simulink model "simTwoLinkFDIbasisComparison"  (R2014b)
settings: Solver=ode45  StartTime=0.0  StopTime=tof  FixedStep=dt  MaxStep=dtmax  RelTol=1e-3
values from neighbouring files (symbols this model uses):
  As = zeros(nofstates,nofstates)    [threeLinkFTC.m]    (also in twoLinkFDIbasisComparison.m; twoLinkFTC.m; twoLinkFTCwAdaptive.m)
  c1 = 0    [robotArmWith2Links.m]    (also in twoLinkFDIbasisComparison.m = 1; twoLinkFTC.m; twoLinkFTCwAdaptive.m)
  c2 = 0    [robotArmWith2Links.m]    (also in twoLinkFDIbasisComparison.m = 1; twoLinkFTC.m; twoLinkFTCwAdaptive.m)
  Dhat0 = zeros(6,1)    [threeLinkFTC.m]    (also in twoLinkFDIbasisComparison.m = zeros(4,1); twoLinkFTC.m = zeros(4,1); twoLinkFTCwAdaptive.m = zeros(4,1))
  dtFc = 1*dtmax    (= 0.001)    [threeLinkFTC.m]    (also in twoLinkFDIbasisComparison.m; twoLinkFTC.m; twoLinkFTCwAdaptive.m)
  epsilontheta = 0.01    [threeLinkFTC.m]    (also in twoLinkFDIbasisComparison.m; twoLinkFTC.m; twoLinkFTCwAdaptive.m)
  fault_gamma = 1    [twoLinkFDIbasisComparison.m]
  fault_taumax = 15    [twoLinkFDIbasisComparison.m]
  faultyArm = 3    [threeLinkFTC.m]    (also in twoLinkFDIbasisComparison.m = 2; twoLinkFTC.m = 2; twoLinkFTCwAdaptive.m = 1)
  g = 9.81    [robotArmWith2Links.m]    (also in threeLinkFTC.m; twoLinkFDIbasisComparison.m; twoLinkFTC.m; twoLinkFTCwAdaptive.m)
  GammaW = 1000    [threeLinkFTC.m]    (also in twoLinkFDIbasisComparison.m; twoLinkFTC.m; twoLinkFTCwAdaptive.m)
  I1 = 8.33e-2    (= 0.0833)    [robotArmWith2Links.m]    (also in threeLinkFTC.m = 0.0833333333333; twoLinkFDIbasisComparison.m = 0.0833333333333; twoLinkFTC.m = 0.0833333333333; twoLinkFTCwAdaptive.m = 0.0833333333333)
  I2 = 8.33e-2    (= 0.0833)    [robotArmWith2Links.m]    (also in threeLinkFTC.m = 0.0833333333333; twoLinkFDIbasisComparison.m = 0.0833333333333; twoLinkFTC.m = 0.0833333333333; twoLinkFTCwAdaptive.m = 0.0833333333333)
  ifault = 2    [threeLinkFTC.m]    (also in twoLinkFDIbasisComparison.m; twoLinkFTC.m; twoLinkFTCwAdaptive.m)
  Kp = wn^2    (= 157.913670417)    [threeLinkFTC.m]    (also in twoLinkFDIbasisComparison.m = 3947.84176044; twoLinkFTC.m = 3947.84176044; twoLinkFTCwAdaptive.m = 3947.84176044)
  Kv = 2*ksi*wn    (= 17.5929188601)    [threeLinkFTC.m]    (also in twoLinkFDIbasisComparison.m = 125.663706144; twoLinkFTC.m = 125.663706144; twoLinkFTCwAdaptive.m = 125.663706144)
  l1 = 1    [robotArmWith2Links.m]    (also in threeLinkFTC.m; twoLinkFDIbasisComparison.m; twoLinkFTC.m; twoLinkFTCwAdaptive.m)
  l2 = 1    [robotArmWith2Links.m]    (also in threeLinkFTC.m; twoLinkFDIbasisComparison.m; twoLinkFTC.m; twoLinkFTCwAdaptive.m)
  lc1 = l1/2    (= 0.5)    [robotArmWith2Links.m]    (also in threeLinkFTC.m; twoLinkFDIbasisComparison.m; twoLinkFTC.m; twoLinkFTCwAdaptive.m)
  lc2 = l2/2    (= 0.5)    [robotArmWith2Links.m]    (also in threeLinkFTC.m; twoLinkFDIbasisComparison.m; twoLinkFTC.m; twoLinkFTCwAdaptive.m)
  m1 = 1    [robotArmWith2Links.m]    (also in threeLinkFTC.m; twoLinkFDIbasisComparison.m; twoLinkFTC.m; twoLinkFTCwAdaptive.m)
  m2 = 1    [robotArmWith2Links.m]    (also in threeLinkFTC.m; twoLinkFDIbasisComparison.m; twoLinkFTC.m; twoLinkFTCwAdaptive.m)
  nCheby = 4    [threeLinkFTC.m]    (also in twoLinkFDIbasisComparison.m; twoLinkFTC.m; twoLinkFTCwAdaptive.m)
  nRBF = length(x1is)*length(x2is)*length(x3is)*length(x4is)    [twoLinkFDIbasisComparison.m]
  Ps = lyap(As(4:6,4:6)',Q)    [threeLinkFTC.m]    (also in twoLinkFDIbasisComparison.m = lyap(As(3:4,3:4)',Q); twoLinkFTC.m = lyap(As(3:4,3:4)',Q); twoLinkFTCwAdaptive.m = lyap(As(3:4,3:4)',Q))
  q0 = [80 20]'*pi/180    [robotArmWith2Links.m]    (also in threeLinkFTC.m = [90 0 0]'*pi/180; twoLinkFDIbasisComparison.m = [90 0]'*pi/180; twoLinkFTC.m = [90 0]'*pi/180; twoLinkFTCwAdaptive.m = [90 0]'*pi/180)
  qdot0 = [0 0]'    [robotArmWith2Links.m]    (also in threeLinkFTC.m = [0 0 0]'*pi/180; twoLinkFDIbasisComparison.m = [0 0]'*pi/180; twoLinkFTC.m = [0 0]'*pi/180; twoLinkFTCwAdaptive.m = [0 0]'*pi/180)
  tfault = 5    [threeLinkFTC.m]    (also in twoLinkFDIbasisComparison.m; twoLinkFTC.m; twoLinkFTCwAdaptive.m = 1)
  visualFlag = 0    [robotArmWith2Links.m]    (also in twoLinkFDIbasisComparison.m; twoLinkFTC.m; twoLinkFTCwAdaptive.m)
  visualizationDataFlag = 1    [robotArmWith2Links.m]    (also in twoLinkFDIbasisComparison.m; twoLinkFTC.m; twoLinkFTCwAdaptive.m)
  W0 = 0    [threeLinkFTC.m]    (also in twoLinkFDIbasisComparison.m; twoLinkFTC.m; twoLinkFTCwAdaptive.m)
  Wbnd = 1000    [threeLinkFTC.m]    (also in twoLinkFDIbasisComparison.m; twoLinkFTC.m; twoLinkFTCwAdaptive.m)
  xhat0 = [q0 ; qdot0]    [threeLinkFTC.m]    (also in twoLinkFDIbasisComparison.m; twoLinkFTC.m; twoLinkFTCwAdaptive.m)
  xu = zeros(nRBF,2)    [twoLinkFDIbasisComparison.m]
undefined symbols (not defined in the file or in its folder): Intmax, Intmin, twolinkplot
libraries: simulink x4, vrlib x4, dspbuff3 x2
(part 1 of 2)
settings Model: Creator=alp.marangoz  LastModifiedBy=alpmarangoz
settings SolverCC: AutoInsertRateTranBlk=on
settings DataIOCC: SignalLoggingSaveFormat=ModelDataLogs
settings OptimizationCC: ExpressionDepthLimit=2147483647
settings DebuggingCC: UnderspecifiedInitializationDetection=Classic  MergeDetectMultiDrivingBlocksExec=none  InheritedTsInSrcMsg=none  CheckMatrixSingularityMsg=error  FcnCallInpInsideContextMsg=UseLocalSettings  StateNameClashWarn=warning
settings GRTTargetCC: CombineOutputUpdateFcns=off  GRTInterface=on

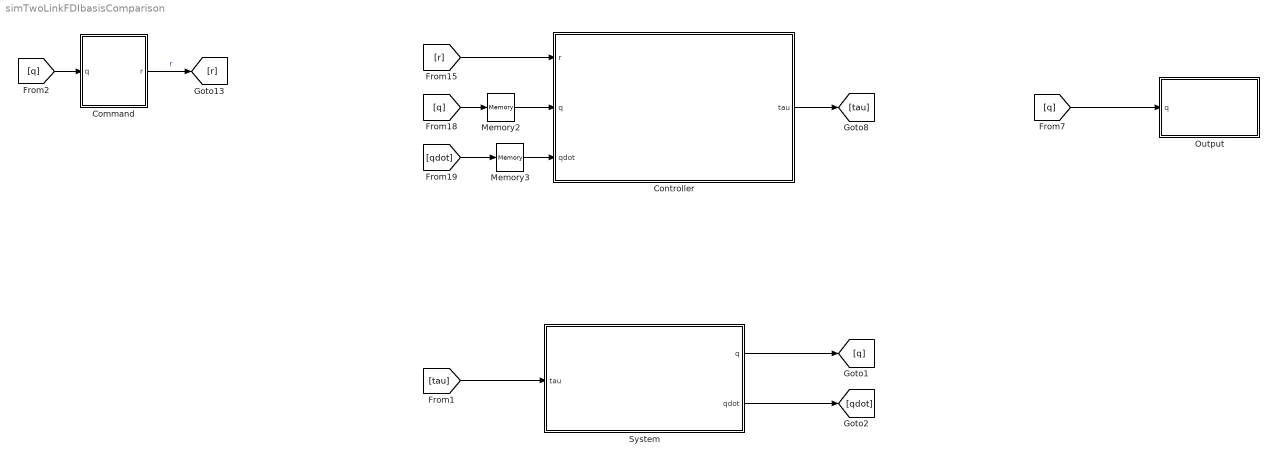
== system simTwoLinkFDIbasisComparison ==
  Command : Subsystem  TreatAsAtomicUnit=on  SystemSampleTime=dtFc
  Controller : Subsystem  TreatAsAtomicUnit=on  SystemSampleTime=dtFc
  Memory2 : Memory  X0=q0  InheritSampleTime=on  LinearizeMemory=on  LinearizeAsDelay=on
  Memory3 : Memory  X0=qdot0  InheritSampleTime=on  LinearizeMemory=on  LinearizeAsDelay=on
  Output : Subsystem  TreatAsAtomicUnit=on
  System : Subsystem  TreatAsAtomicUnit=on
  wires:
  Command/1(r) -> [r]  "r"
  [r] -> Controller/1(r)
  Controller/1(tau) -> [tau]
  [q] -> Output/1(q)
  [tau] -> System/1(tau)
  [q] -> Memory2/1
  [qdot] -> Memory3/1
  System/1(q) -> [q]
  System/2(qdot) -> [qdot]
  [q] -> Command/1(q)
  Memory2/1 -> Controller/2(q)
  Memory3/1 -> Controller/3(qdot)

== system simTwoLinkFDIbasisComparison/Command ==
  q : Inport
  Add1 : Sum  Inputs=-+
  From Workspace : FromWorkspace  VariableName=r  Interpolate=off  OutputAfterFinalValue=Setting to zero
  Memory2 : Memory  X0=q0  InheritSampleTime=on  LinearizeMemory=on  LinearizeAsDelay=on
  Reshape1 : Reshape  OutputDimensionality=Column vector (2-D)
  Terminator1 : Terminator
  r : Outport  InitialOutput=0
  wires:
  From Workspace/1 -> Reshape1/1
  Reshape1/1 -> r/1, [r]  "r"
  [r] -> Add1/2
  Add1/1 -> Terminator1/1  "e"
  [q] -> Add1/1  "q"
  q/1 -> Memory2/1  "q"
  Memory2/1 -> [q]

== system simTwoLinkFDIbasisComparison/Controller ==
  r : Inport
  q : Inport  Port=2
  qdot : Inport  Port=3
  Disturbance Estimator : Subsystem
  Gain : Gain  Gain=-1
  Get System Parameters : Subsystem
  Nominal Controller : Subsystem
  Terminator1 : Terminator
  Terminator2 : Terminator
  tau : Outport
  wires:
  r/1 -> [r]  "r"
  qdot/1 -> [qdot]  "qdot"
  q/1 -> [q]  "q"
  [tau] -> tau/1  "tau"
  [q] -> Get System Parameters/1(q)
  Nominal Controller/1(tau) -> [tau]
  [r] -> Nominal Controller/1(r)
  [H] -> Nominal Controller/4(H)
  [Phi] -> Nominal Controller/5(Phi)
  [qdot] -> Get System Parameters/2(qdot)
  Get System Parameters/1(H) -> [H]
  Get System Parameters/2(Phi) -> [Phi]
  Get System Parameters/3(Cprime) -> [Cp]
  [q] -> Disturbance Estimator/1(q)
  [qdot] -> Disturbance Estimator/2(qdot)
  [H] -> Disturbance Estimator/4(H)
  [Cp] -> Disturbance Estimator/5(Cp)
  [G] -> Disturbance Estimator/6(G)
  Disturbance Estimator/1(xhat) -> Terminator1/1  "xhat"
  Disturbance Estimator/2(Dhat) -> [Dhat]
  [qdot] -> Nominal Controller/3(qdot)
  [q] -> Nominal Controller/2(q)
  [tau] -> Disturbance Estimator/3(tau)
  Get System Parameters/4(G) -> [G]
  Gain/1 -> Terminator2/1  "Dhat"
  [Dhat] -> Gain/1

== system simTwoLinkFDIbasisComparison/Output ==
  q : Inport
  Constant1 : Constant  Value=visualFlag
  Constant3 : Constant  Value=visualizationDataFlag
  Demux4 : Demux  Outputs=2
  two link visualization : Subsystem
  visualization data out : Subsystem  TreatAsAtomicUnit=on
  wires:
  Constant1/1 -> two link visualization/Enable
  Demux4/1 -> two link visualization/1(tht1 [|rad])
  Demux4/2 -> two link visualization/2(tht2 [rad])
  Constant3/1 -> visualization data out/Enable
  q/1 -> visualization data out/1(tht), Demux4/1

== system simTwoLinkFDIbasisComparison/System ==
  tau : Inport
  Fault Insertion : Subsystem
  Integration : Subsystem  TreatAsAtomicUnit=on
  Memory2 : Memory  X0=q0  InheritSampleTime=on  LinearizeMemory=on  LinearizeAsDelay=on
  Memory4 : Memory  X0=qdot0  InheritSampleTime=on  LinearizeMemory=on  LinearizeAsDelay=on
  Reshape5 : Reshape  OutputDimensionality=Column vector (2-D)
  System Parameters : Subsystem
  q : Outport
  qdot : Outport  Port=2
  wires:
  System Parameters/1(H) -> [H]
  System Parameters/2(Phi) -> [Phi]
  [q] -> Memory2/1
  [qdot] -> Memory4/1
  tau/1 -> Reshape5/1  "tau"
  Reshape5/1 -> [tau]  "tau"
  [q] -> q/1  "q"
  [qdot] -> qdot/1  "qdot"
  [tau] -> Fault Insertion/1(tau)
  [Phi] -> Fault Insertion/2(Phi)
  Fault Insertion/2(lockJoint) -> [lockJoint]
  Memory4/1 -> System Parameters/2(qdot)
  [H] -> Integration/1(H)
  [C] -> Integration/2(C)
  [tau] -> Integration/5(tau)
  [lockJoint] -> Integration/6(lockJoint)
  System Parameters/3(C) -> [C]
  System Parameters/4(G) -> [G]
  [G] -> Integration/3(G)
  [F] -> Integration/4(F)
  Integration/1(q) -> [q]
  Integration/2(qdot) -> [qdot]
  Memory2/1 -> System Parameters/1(q)
  Fault Insertion/1(F) -> [F]

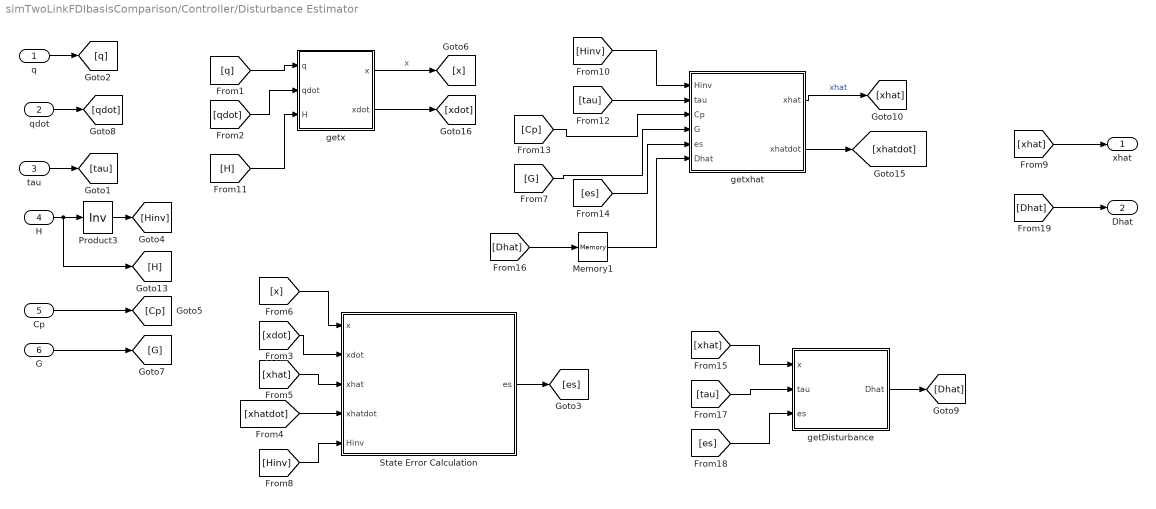
== system simTwoLinkFDIbasisComparison/Controller/Disturbance Estimator ==
  q : Inport
  qdot : Inport  Port=2
  tau : Inport  Port=3
  H : Inport  Port=4
  Cp : Inport  Port=5
  G : Inport  Port=6
  Memory1 : Memory  X0=Dhat0  InheritSampleTime=on  LinearizeMemory=on
  Product3 : Product  Inputs=/  Multiplication=Matrix(*)  RndMeth=Zero
  State Error Calculation : Subsystem
  getDisturbance : Subsystem
  getx : Subsystem
  getxhat : Subsystem
  xhat : Outport
  Dhat : Outport  Port=2
  wires:
  getx/2(xdot) -> [xdot]
  [qdot] -> getx/2(qdot)
  [q] -> getx/1(q)
  Cp/1 -> [Cp]
  Product3/1 -> [Hinv]
  H/1 -> [H], Product3/1
  tau/1 -> [tau]
  [xhat] -> xhat/1
  q/1 -> [q]
  qdot/1 -> [qdot]
  getx/1(x) -> [x]  "x"
  [H] -> getx/3(H)
  [Hinv] -> getxhat/1(Hinv)
  [tau] -> getxhat/2(tau)
  [Cp] -> getxhat/3(Cp)
  [es] -> getxhat/5(es)
  [Dhat] -> Memory1/1
  G/1 -> [G]
  getxhat/1(xhat) -> [xhat]  "xhat"
  getxhat/2(xhatdot) -> [xhatdot]
  [x] -> State Error Calculation/1(x)
  [xdot] -> State Error Calculation/2(xdot)
  [xhat] -> State Error Calculation/3(xhat)
  [xhatdot] -> State Error Calculation/4(xhatdot)
  [Hinv] -> State Error Calculation/5(Hinv)
  State Error Calculation/1(es) -> [es]
  [xhat] -> getDisturbance/1(x)
  [tau] -> getDisturbance/2(tau)
  [es] -> getDisturbance/3(es)
  getDisturbance/1(Dhat) -> [Dhat]
  [Dhat] -> Dhat/1
  Memory1/1 -> getxhat/6(Dhat)
  [G] -> getxhat/4(G)

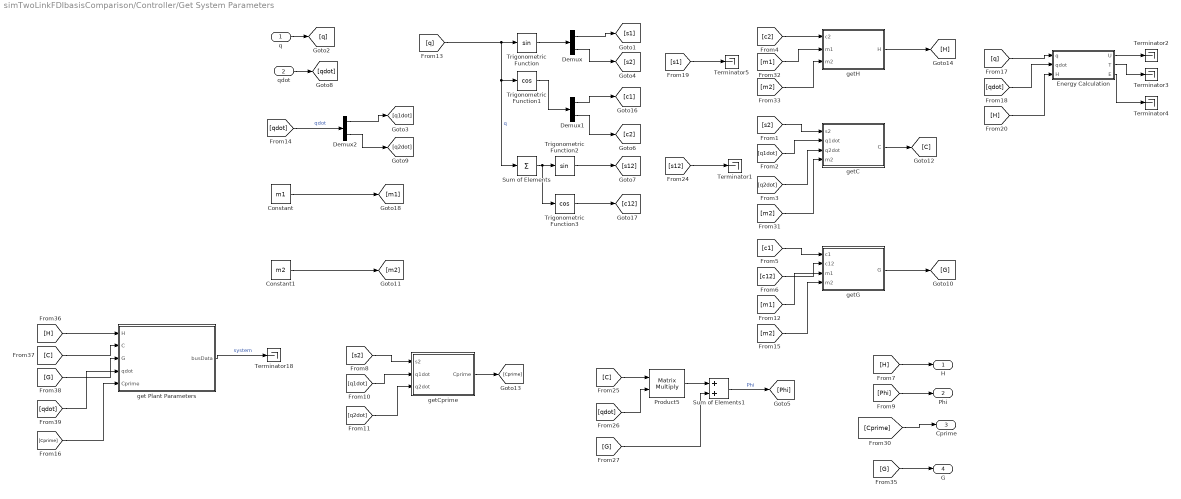
== system simTwoLinkFDIbasisComparison/Controller/Get System Parameters ==
  q : Inport
  qdot : Inport  Port=2
  Constant : Constant  Value=m1
  Constant1 : Constant  Value=m2
  Demux : Demux  Outputs=2
  Demux1 : Demux  Outputs=2
  Demux2 : Demux  Outputs=2
  Energy Calculation : Subsystem
  Product5 : Product  Multiplication=Matrix(*)  RndMeth=Zero
  Sum of Elements : Sum  Inputs=+
  Sum of Elements1 : Sum
  Terminator{1..5,18} (6 alike) : Terminator
  Trigonometric Function : Trigonometry
  Trigonometric Function1 : Trigonometry  Operator=cos
  Trigonometric Function2 : Trigonometry
  Trigonometric Function3 : Trigonometry  Operator=cos
  get Plant Parameters : Subsystem
  getC : Subsystem
  getCprime : Subsystem
  getG : Subsystem
  getH : Subsystem
  H : Outport
  Phi : Outport  Port=2
  Cprime : Outport  Port=3
  G : Outport  Port=4
  wires:
  q/1 -> [q]
  qdot/1 -> [qdot]
  [q] -> Trigonometric Function/1, Trigonometric Function1/1, Sum of Elements/1  "q"
  Trigonometric Function/1 -> Demux/1
  Demux/1 -> [s1]
  Demux/2 -> [s2]
  Demux1/1 -> [c1]
  Demux1/2 -> [c2]
  Trigonometric Function1/1 -> Demux1/1
  Sum of Elements/1 -> Trigonometric Function2/1, Trigonometric Function3/1
  Trigonometric Function2/1 -> [s12]
  [qdot] -> Demux2/1  "qdot"
  Demux2/1 -> [q1dot]
  Demux2/2 -> [q2dot]
  Trigonometric Function3/1 -> [c12]
  [s12] -> Terminator1/1
  [s1] -> Terminator5/1
  [c2] -> getH/1(c2)
  [s2] -> getC/1(s2)
  [q1dot] -> getC/2(q1dot)
  [q2dot] -> getC/3(q2dot)
  getH/1(H) -> [H]
  getC/1(C) -> [C]
  [c1] -> getG/1(c1)
  [c12] -> getG/2(c12)
  getG/1(G) -> [G]
  [q] -> Energy Calculation/1(q)
  [qdot] -> Energy Calculation/2(qdot)
  Energy Calculation/1(U) -> Terminator2/1
  Energy Calculation/2(T) -> Terminator3/1
  Energy Calculation/3(E) -> Terminator4/1
  [H] -> Energy Calculation/3(H)
  [C] -> Product5/1
  [qdot] -> Product5/2
  Product5/1 -> Sum of Elements1/1
  [G] -> Sum of Elements1/2
  Sum of Elements1/1 -> [Phi]  "Phi"
  [H] -> H/1
  [Phi] -> Phi/1
  [s2] -> getCprime/1(s2)
  [q1dot] -> getCprime/2(q1dot)
  [q2dot] -> getCprime/3(q2dot)
  getCprime/1(Cprime) -> [Cprime]
  [Cprime] -> Cprime/1
  [m1] -> getG/3(m1)
  [m2] -> getG/4(m2)
  [m2] -> getC/4(m2)
  [m1] -> getH/2(m1)
  [m2] -> getH/3(m2)
  Constant/1 -> [m1]
  Constant1/1 -> [m2]
  [G] -> G/1
  get Plant Parameters/1(busData) -> Terminator18/1  "system"
  [C] -> get Plant Parameters/2(C)
  [H] -> get Plant Parameters/1(H)
  [G] -> get Plant Parameters/3(G)
  [qdot] -> get Plant Parameters/4(qdot)
  [Cprime] -> get Plant Parameters/5(Cprime)

== system simTwoLinkFDIbasisComparison/Controller/Nominal Controller ==
  r : Inport
  q : Inport  Port=2
  qdot : Inport  Port=3
  H : Inport  Port=4
  Phi : Inport  Port=5
  FBL Controller : Subsystem
  Saturation : Saturate  UpperLimit=2000  LowerLimit=-2000
  tau : Outport
  wires:
  r/1 -> [r]  "r"
  Phi/1 -> [Phi]
  H/1 -> [H]
  [tau] -> Saturation/1  "tau"
  [r] -> FBL Controller/1(r)
  [H] -> FBL Controller/4(H)
  [Phi] -> FBL Controller/5(Phi)
  Saturation/1 -> tau/1
  FBL Controller/1(tau) -> [tau]
  q/1 -> [q]
  qdot/1 -> [qdot]
  [qdot] -> FBL Controller/3(qdot)
  [q] -> FBL Controller/2(q)

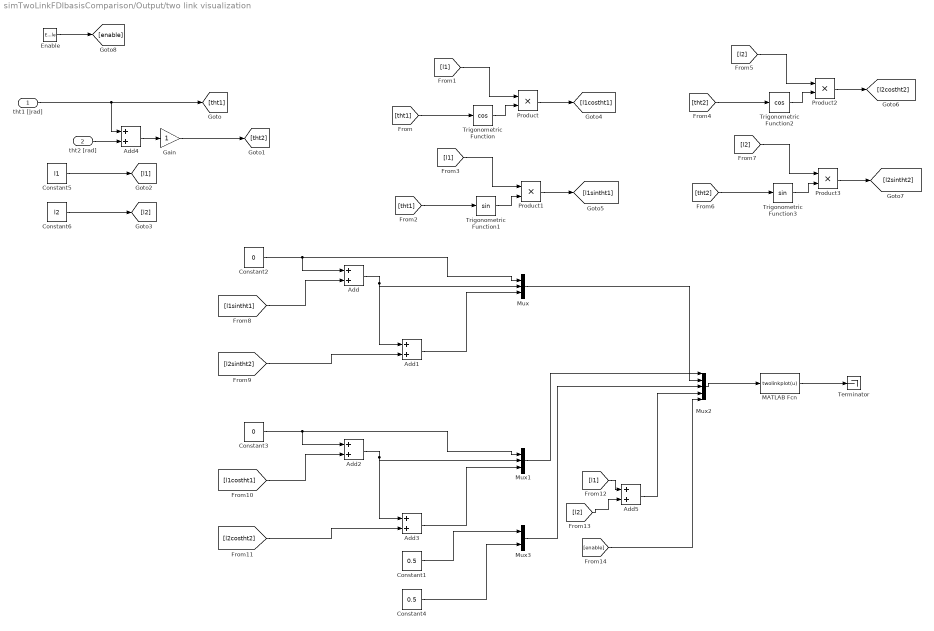
== system simTwoLinkFDIbasisComparison/Output/two link visualization ==
  tht1 [|rad] : Inport
  tht2 [rad] : Inport  Port=2
  Enable : EnablePort  PropagateVarSize=During execution  ShowOutputPort=on
  Add{,1..5} (6 alike) : Sum
  Constant1 : Constant  Value=0.5
  Constant2 : Constant  Value=0
  Constant3 : Constant  Value=0
  Constant4 : Constant  Value=0.5
  Constant5 : Constant  Value=l1  VectorParams1D=off
  Constant6 : Constant  Value=l2  VectorParams1D=off
  Gain : Gain
  MATLAB Fcn : MATLABFcn  MATLABFcn=twolinkplot(u)
  Mux : Mux  Inputs=3
  Mux1 : Mux  Inputs=3
  Mux2 : Mux  Inputs=5
  Mux3 : Mux  Inputs=2
  Product{,1..3} (4 alike) : Product  RndMeth=Zero
  Terminator : Terminator
  Trigonometric Function : Trigonometry  Operator=cos
  Trigonometric Function1 : Trigonometry
  Trigonometric Function2 : Trigonometry  Operator=cos
  Trigonometric Function3 : Trigonometry
  wires:
  [tht1] -> Trigonometric Function/1
  Constant5/1 -> [l1]
  Constant6/1 -> [l2]
  [l1] -> Product/1
  Trigonometric Function/1 -> Product/2
  Product/1 -> [l1costht1]
  [tht1] -> Trigonometric Function1/1
  [l1] -> Product1/1
  Trigonometric Function1/1 -> Product1/2
  Product1/1 -> [l1sintht1]
  [tht2] -> Trigonometric Function2/1
  [l2] -> Product2/1
  Trigonometric Function2/1 -> Product2/2
  Product2/1 -> [l2costht2]
  [tht2] -> Trigonometric Function3/1
  [l2] -> Product3/1
  Trigonometric Function3/1 -> Product3/2
  Product3/1 -> [l2sintht2]
  Constant2/1 -> Add/1, Mux/1
  [l1sintht1] -> Add/2
  Add/1 -> Add1/1, Mux/2
  [l2sintht2] -> Add1/2
  Add1/1 -> Mux/3
  Constant3/1 -> Mux1/1, Add2/1
  [l1costht1] -> Add2/2
  Add2/1 -> Mux1/2, Add3/1
  [l2costht2] -> Add3/2
  Add3/1 -> Mux1/3
  Mux2/1 -> MATLAB Fcn/1
  MATLAB Fcn/1 -> Terminator/1
  tht2 [rad]/1 -> Add4/2
  Gain/1 -> [tht2]
  Add4/1 -> Gain/1
  [l1] -> Add5/1
  [l2] -> Add5/2
  Enable/1 -> [enable]
  Constant1/1 -> Mux3/1
  Constant4/1 -> Mux3/2
  Mux3/1 -> Mux2/3
  Add5/1 -> Mux2/4
  [enable] -> Mux2/5
  tht1 [|rad]/1 -> Add4/1, [tht1]
  Mux1/1 -> Mux2/1
  Mux/1 -> Mux2/2

== system simTwoLinkFDIbasisComparison/Output/visualization data out ==
  tht : Inport
  Enable : EnablePort  PropagateVarSize=During execution
  To Workspace : ToWorkspace  VariableName=thetaForVisualization  SaveFormat=Structure With Time  SampleTime=-1
  wires:
  tht/1 -> To Workspace/1

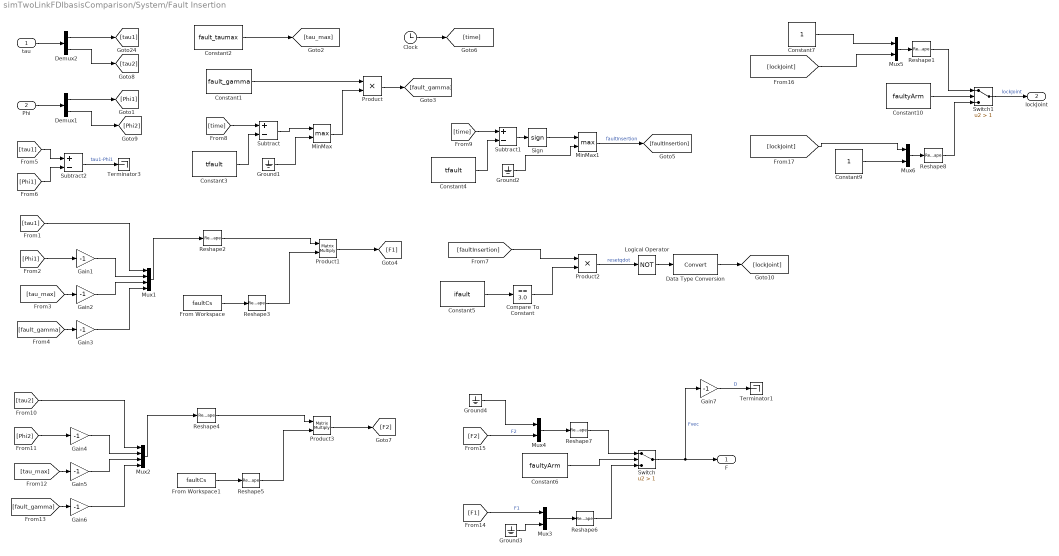
== system simTwoLinkFDIbasisComparison/System/Fault Insertion ==
  tau : Inport
  Phi : Inport  Port=2
  Clock : Clock
  Compare To Constant : simulink/Logic and Bit Operations/Compare To Constant  relop===  const=3.0  OutDataTypeStr=uint8  ZeroCross=off
  Constant1 : Constant  Value=fault_gamma
  Constant10 : Constant  Value=faultyArm  VectorParams1D=off
  Constant2 : Constant  Value=fault_taumax
  Constant3 : Constant  Value=tfault
  Constant4 : Constant  Value=tfault
  Constant5 : Constant  Value=ifault
  Constant6 : Constant  Value=faultyArm  VectorParams1D=off
  Constant7 : Constant
  Constant9 : Constant
  Data Type Conversion : DataTypeConversion
  Demux1 : Demux  Outputs=2
  Demux2 : Demux  Outputs=2
  From Workspace : FromWorkspace  VariableName=faultCs  Interpolate=off  OutputAfterFinalValue=Setting to zero
  From Workspace1 : FromWorkspace  VariableName=faultCs  Interpolate=off  OutputAfterFinalValue=Setting to zero
  Gain{1..7} (7 alike) : Gain  Gain=-1
  Ground{1..4} (4 alike) : Ground
  Logical Operator : Logic  Operator=NOT  AllPortsSameDT=off  OutDataTypeStr=boolean
  MinMax : MinMax  Function=max  Inputs=2
  MinMax1 : MinMax  Function=max  Inputs=2
  Mux1 : Mux
  Mux2 : Mux
  Mux{3..6} (4 alike) : Mux  Inputs=2
  Product : Product  RndMeth=Zero
  Product1 : Product  Multiplication=Matrix(*)  RndMeth=Zero
  Product2 : Product  RndMeth=Zero
  Product3 : Product  Multiplication=Matrix(*)  RndMeth=Zero
  Reshape{1,3,5..8} (6 alike) : Reshape  OutputDimensionality=Column vector (2-D)
  Reshape2 : Reshape  OutputDimensionality=Row vector (2-D)
  Reshape4 : Reshape  OutputDimensionality=Row vector (2-D)
  Sign : Signum
  Subtract : Sum  Inputs=+-
  Subtract1 : Sum  Inputs=+-
  Subtract2 : Sum  Inputs=+-
  Switch : Switch  Criteria=u2 > Threshold  Threshold=1  ZeroCross=off
  Switch1 : Switch  Criteria=u2 > Threshold  Threshold=1  ZeroCross=off
  Terminator1 : Terminator
  Terminator3 : Terminator
  F : Outport
  lockJoint : Outport  Port=2
  wires:
  tau/1 -> Demux2/1
  Phi/1 -> Demux1/1
  Demux2/1 -> [tau1]
  Demux2/2 -> [tau2]
  Demux1/1 -> [Phi1]
  Demux1/2 -> [Phi2]
  Constant2/1 -> [tau_max]
  [tau1] -> Mux1/1
  [Phi1] -> Gain1/1
  [tau_max] -> Gain2/1
  [fault_gamma] -> Gain3/1
  Mux1/1 -> Reshape2/1
  Reshape2/1 -> Product1/1
  [time] -> Subtract/1
  Constant3/1 -> Subtract/2
  Subtract/1 -> MinMax/1
  Ground1/1 -> MinMax/2
  Constant1/1 -> Product/1
  MinMax/1 -> Product/2
  Product/1 -> [fault_gamma]
  From Workspace/1 -> Reshape3/1
  Reshape3/1 -> Product1/2
  Product1/1 -> [F1]
  Gain1/1 -> Mux1/2
  Gain2/1 -> Mux1/3
  Gain3/1 -> Mux1/4
  [time] -> Subtract1/1
  Constant4/1 -> Subtract1/2
  Subtract1/1 -> Sign/1
  Ground2/1 -> MinMax1/2
  Sign/1 -> MinMax1/1
  MinMax1/1 -> [faultInsertion]  "faultInsertion"
  [tau1] -> Subtract2/1
  [Phi1] -> Subtract2/2
  Subtract2/1 -> Terminator3/1  "tau1-Phi1"
  Constant5/1 -> Compare To Constant/1
  [faultInsertion] -> Product2/1
  Compare To Constant/1 -> Product2/2
  Product2/1 -> Logical Operator/1  "resetqdot"
  Logical Operator/1 -> Data Type Conversion/1
  Clock/1 -> [time]
  [tau2] -> Mux2/1
  [Phi2] -> Gain4/1
  [tau_max] -> Gain5/1
  [fault_gamma] -> Gain6/1
  Mux2/1 -> Reshape4/1
  Reshape4/1 -> Product3/1
  From Workspace1/1 -> Reshape5/1
  Reshape5/1 -> Product3/2
  Product3/1 -> [F2]
  Gain4/1 -> Mux2/2
  Gain5/1 -> Mux2/3
  Gain6/1 -> Mux2/4
  Mux3/1 -> Reshape6/1
  Ground3/1 -> Mux3/2
  [F1] -> Mux3/1  "F1"
  Mux4/1 -> Reshape7/1
  [F2] -> Mux4/2  "F2"
  Ground4/1 -> Mux4/1
  Switch/1 -> Gain7/1, F/1  "Fvec"
  Reshape7/1 -> Switch/1
  Reshape6/1 -> Switch/3
  Constant6/1 -> Switch/2
  Mux5/1 -> Reshape1/1
  Data Type Conversion/1 -> [lockJoint]
  Switch1/1 -> lockJoint/1  "lockJoint"
  Mux6/1 -> Reshape8/1
  Constant9/1 -> Mux6/2
  [lockJoint] -> Mux6/1
  Constant7/1 -> Mux5/1
  [lockJoint] -> Mux5/2
  Reshape1/1 -> Switch1/1
  Constant10/1 -> Switch1/2
  Reshape8/1 -> Switch1/3
  Gain7/1 -> Terminator1/1  "D"

== system simTwoLinkFDIbasisComparison/System/Integration ==
  H : Inport
  C : Inport  Port=2
  G : Inport  Port=3
  F : Inport  Port=4
  tau : Inport  Port=5
  lockJoint : Inport  Port=6
  Add : Sum  Inputs=+--
  Constant1 : Constant  Value=2*pi
  Integrator2 : Integrator  InitialCondition=qdot0
  Integrator3 : Integrator  InitialCondition=q0
  Math Function1 : Math  Operator=rem  SaturateOnIntegerOverflow=on
  Product1 : Product  RndMeth=Zero
  Product3 : Product  RndMeth=Zero
  Product4 : Product  Multiplication=Matrix(*)  RndMeth=Zero
  Product5 : Product  Multiplication=Matrix(*)  RndMeth=Zero
  Product6 : Product  Multiplication=Matrix(*)  RndMeth=Zero
  Product7 : Product  Inputs=/  Multiplication=Matrix(*)  RndMeth=Zero
  Reshape : Reshape  OutputDimensionality=Column vector (2-D)
  Reshape3 : Reshape  OutputDimensionality=Column vector (2-D)
  Sum : Sum  Inputs=|+-
  q : Outport
  qdot : Outport  Port=2
  wires:
  lockJoint/1 -> [lockJoint]
  tau/1 -> [tau]
  F/1 -> [F]
  C/1 -> [C]
  H/1 -> Product7/1
  [qdot] -> qdot/1  "qdot"
  [q] -> q/1  "q"
  G/1 -> [G]
  [G] -> Add/2
  [Hinv] -> Product4/1
  Add/1 -> Product4/2
  Product4/1 -> Sum/1
  [Hinv] -> Product5/1
  [C] -> Product5/2
  Product5/1 -> Product6/1
  Product6/1 -> Sum/2
  Integrator3/1 -> Reshape3/1
  Reshape/1 -> Product6/2, Integrator3/1, [qdot]
  Reshape3/1 -> Math Function1/1
  Product7/1 -> [Hinv]
  [tau] -> Add/1
  Constant1/1 -> Math Function1/2
  Math Function1/1 -> [q]  "qr"
  Sum/1 -> Product3/2
  Product3/1 -> Integrator2/1  "qddot"
  [F] -> Add/3
  [lockJoint] -> Product3/1, Product1/1
  Integrator2/1 -> Product1/2
  Product1/1 -> Reshape/1  "qdot"

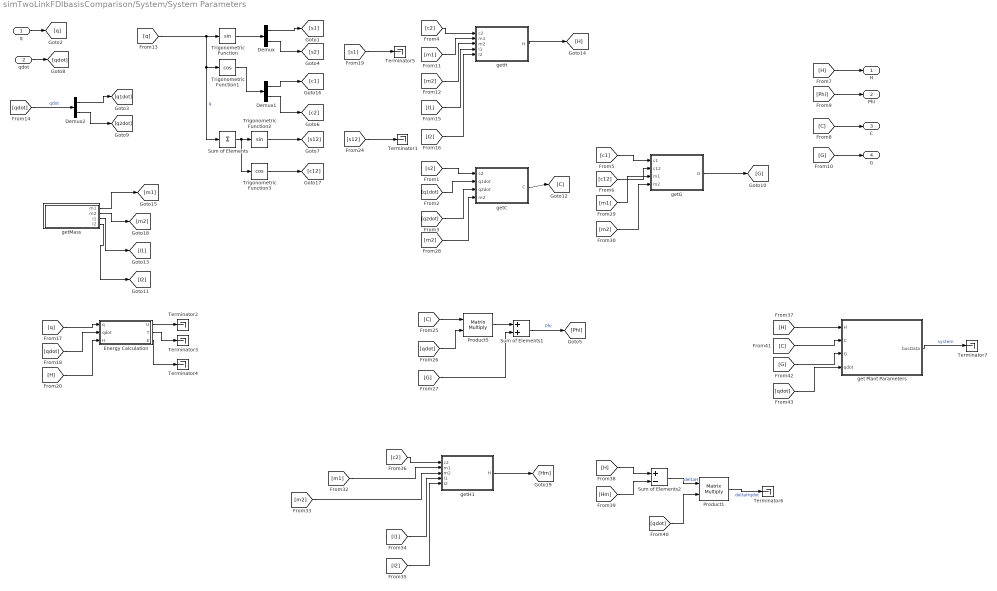
== system simTwoLinkFDIbasisComparison/System/System Parameters ==
  q : Inport
  qdot : Inport  Port=2
  Demux : Demux  Outputs=2
  Demux1 : Demux  Outputs=2
  Demux2 : Demux  Outputs=2
  Energy Calculation : Subsystem
  Product1 : Product  Multiplication=Matrix(*)  RndMeth=Zero
  Product5 : Product  Multiplication=Matrix(*)  RndMeth=Zero
  Sum of Elements : Sum  Inputs=+
  Sum of Elements1 : Sum
  Sum of Elements2 : Sum  Inputs=+-
  Terminator{1..7} (7 alike) : Terminator
  Trigonometric Function : Trigonometry
  Trigonometric Function1 : Trigonometry  Operator=cos
  Trigonometric Function2 : Trigonometry
  Trigonometric Function3 : Trigonometry  Operator=cos
  get Plant Parameters : Subsystem
  getC : Subsystem
  getG : Subsystem
  getH : Subsystem
  getH1 : Subsystem
  getMass : Subsystem
  H : Outport
  Phi : Outport  Port=2
  C : Outport  Port=3
  G : Outport  Port=4
  wires:
  q/1 -> [q]
  qdot/1 -> [qdot]
  [q] -> Trigonometric Function/1, Trigonometric Function1/1, Sum of Elements/1  "q"
  Trigonometric Function/1 -> Demux/1
  Demux/1 -> [s1]
  Demux/2 -> [s2]
  Demux1/1 -> [c1]
  Demux1/2 -> [c2]
  Trigonometric Function1/1 -> Demux1/1
  Sum of Elements/1 -> Trigonometric Function2/1, Trigonometric Function3/1
  Trigonometric Function2/1 -> [s12]
  [qdot] -> Demux2/1  "qdot"
  Demux2/1 -> [q1dot]
  Demux2/2 -> [q2dot]
  Trigonometric Function3/1 -> [c12]
  [s12] -> Terminator1/1
  [s1] -> Terminator5/1
  [c2] -> getH/1(c2)
  [s2] -> getC/1(s2)
  [q1dot] -> getC/2(q1dot)
  [q2dot] -> getC/3(q2dot)
  getH/1(H) -> [H]
  getC/1(C) -> [C]
  [c1] -> getG/1(c1)
  [c12] -> getG/2(c12)
  getG/1(G) -> [G]
  [q] -> Energy Calculation/1(q)
  [qdot] -> Energy Calculation/2(qdot)
  Energy Calculation/1(U) -> Terminator2/1
  Energy Calculation/2(T) -> Terminator3/1
  Energy Calculation/3(E) -> Terminator4/1
  [H] -> Energy Calculation/3(H)
  [C] -> Product5/1
  [qdot] -> Product5/2
  Product5/1 -> Sum of Elements1/1
  [G] -> Sum of Elements1/2
  Sum of Elements1/1 -> [Phi]  "Phi"
  [H] -> H/1
  [Phi] -> Phi/1
  [C] -> C/1
  [G] -> G/1
  [m1] -> getH/2(m1)
  [m2] -> getH/3(m2)
  [I1] -> getH/4(I1)
  [I2] -> getH/5(I2)
  [m2] -> getC/4(m2)
  [m1] -> getG/3(m1)
  [m2] -> getG/4(m2)
  getMass/1(m1) -> [m1]
  getMass/2(m2) -> [m2]
  getMass/3(I1) -> [I1]
  getMass/4(I2) -> [I2]
  [c2] -> getH1/1(c2)
  getH1/1(H) -> [Hm]
  [I1] -> getH1/4(I1)
  [I2] -> getH1/5(I2)
  [H] -> Sum of Elements2/1
  [Hm] -> Sum of Elements2/2
  Sum of Elements2/1 -> Product1/1  "deltaH"
  [qdot] -> Product1/2
  Product1/1 -> Terminator6/1  "deltaHqdot"
  [m2] -> getH1/3(m2)
  [m1] -> getH1/2(m1)
  get Plant Parameters/1(busData) -> Terminator7/1  "system"
  [C] -> get Plant Parameters/2(C)
  [H] -> get Plant Parameters/1(H)
  [G] -> get Plant Parameters/3(G)
  [qdot] -> get Plant Parameters/4(qdot)

== system simTwoLinkFDIbasisComparison/Controller/Disturbance Estimator/State Error Calculation ==
  x : Inport
  xdot : Inport  Port=2
  xhat : Inport  Port=3
  xhatdot : Inport  Port=4
  Hinv : Inport  Port=5
  Add : Sum  Inputs=+-
  Add1 : Sum  Inputs=+-
  Discrete Derivative1 : simulink/Discrete/Discrete Derivative  gainval=1.0  ICPrevScaledInput=0.0  InputProcessing=Inherited  OutMin=[]  OutMax=[]  OutDataType=fixdt(1, 16)  OutScaling=2^-10  RndMeth=Round  DoSatur=off
  Memory1 : Memory  X0=xhat0  InheritSampleTime=on  LinearizeMemory=on  LinearizeAsDelay=on
  Memory4 : Memory  X0=xhat0  InheritSampleTime=on  LinearizeMemory=on  LinearizeAsDelay=on
  Product6 : Product  Multiplication=Matrix(*)  RndMeth=Zero
  Reshape1 : Reshape  OutputDimensionality=Column vector (2-D)
  Reshape2 : Reshape  OutputDimensionality=Column vector (2-D)
  Reshape3 : Reshape  OutputDimensionality=Column vector (2-D)
  Saturation : Saturate  UpperLimit=10  LowerLimit=-10  ZeroCross=off
  Terminator{1..4} (4 alike) : Terminator
  "[1 2]" : Selector  NumberOfDimensions=2  InputPortWidth=3  IndexOptions=Index vector (dialog),Index vector (dialog)  Indices=[1 2],1  OutputSizes=1,1
  "[3 4]" : Selector  NumberOfDimensions=2  InputPortWidth=3  IndexOptions=Index vector (dialog),Index vector (dialog)  Indices=[3 4],1  OutputSizes=1,1
  es : Outport
  wires:
  [Hinv] -> Product6/1
  xdot/1 -> [xdot]
  x/1 -> [x]
  Saturation/1 -> [esdot]  "esdotflt"
  Discrete Derivative1/1 -> Saturation/1  "esdot"
  Reshape2/1 -> [es], Discrete Derivative1/1
  [xhat] -> Memory4/1
  [x] -> Add/2
  Add/1 -> Reshape2/1  "es"
  Memory4/1 -> Add/1
  xhat/1 -> [xhat]
  xhatdot/1 -> [xhatdot]
  Hinv/1 -> [Hinv]
  [xhatdot] -> Memory1/1
  [xdot] -> Add1/2
  Add1/1 -> Reshape1/1  "esdot2"
  Memory1/1 -> Add1/1
  [esdot] -> Terminator3/1
  [es] -> es/1
  [xhat] -> Reshape3/1
  Reshape3/1 -> "[1 2]"/1, "[3 4]"/1
  "[3 4]"/1 -> Product6/2
  "[1 2]"/1 -> Terminator2/1  "qhat"
  Product6/1 -> Terminator1/1  "qhatdot"
  Reshape1/1 -> Terminator4/1

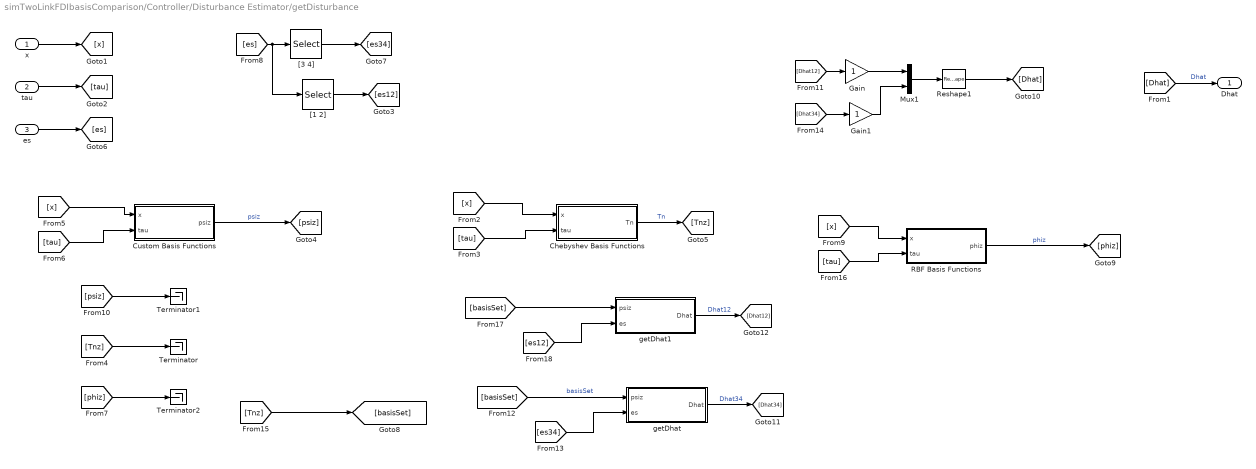
== system simTwoLinkFDIbasisComparison/Controller/Disturbance Estimator/getDisturbance ==
  x : Inport
  tau : Inport  Port=2
  es : Inport  Port=3
  Chebyshev Basis Functions : Subsystem
  Custom Basis Functions : Subsystem
  Gain : Gain
  Gain1 : Gain
  Mux1 : Mux  Inputs=2
  RBF Basis Functions : Subsystem
  Reshape1 : Reshape  OutputDimensionality=Column vector (2-D)
  Terminator : Terminator
  Terminator1 : Terminator
  Terminator2 : Terminator
  "[1 2]" : Selector  NumberOfDimensions=2  InputPortWidth=3  IndexOptions=Index vector (dialog),Index vector (dialog)  Indices=[1 2],1  OutputSizes=1,1
  "[3 4]" : Selector  NumberOfDimensions=2  InputPortWidth=3  IndexOptions=Index vector (dialog),Index vector (dialog)  Indices=[3 4],1  OutputSizes=1,1
  getDhat : Subsystem  TreatAsAtomicUnit=on
  getDhat1 : Subsystem  TreatAsAtomicUnit=on
  Dhat : Outport
  wires:
  [Dhat] -> Dhat/1  "Dhat"
  x/1 -> [x]
  tau/1 -> [tau]
  es/1 -> [es]
  [es] -> "[1 2]"/1, "[3 4]"/1
  "[3 4]"/1 -> [es34]
  [Dhat12] -> Gain/1
  Mux1/1 -> Reshape1/1
  Reshape1/1 -> [Dhat]
  [Dhat34] -> Gain1/1
  [basisSet] -> getDhat/1(psiz)  "basisSet"
  [es34] -> getDhat/2(es)
  getDhat/1(Dhat) -> [Dhat34]  "Dhat34"
  Gain/1 -> Mux1/1
  Gain1/1 -> Mux1/2
  [x] -> Custom Basis Functions/1(x)
  [tau] -> Custom Basis Functions/2(tau)
  Custom Basis Functions/1(psiz) -> [psiz]  "psiz"
  Chebyshev Basis Functions/1(Tn) -> [Tnz]  "Tn"
  [x] -> Chebyshev Basis Functions/1(x)
  [tau] -> Chebyshev Basis Functions/2(tau)
  [Tnz] -> Terminator/1
  [psiz] -> Terminator1/1
  [Tnz] -> [basisSet]
  RBF Basis Functions/1(phiz) -> [phiz]  "phiz"
  [phiz] -> Terminator2/1
  [tau] -> RBF Basis Functions/2(tau)
  [x] -> RBF Basis Functions/1(x)
  [basisSet] -> getDhat1/1(psiz)
  [es12] -> getDhat1/2(es)
  getDhat1/1(Dhat) -> [Dhat12]  "Dhat12"
  "[1 2]"/1 -> [es12]

== system simTwoLinkFDIbasisComparison/Controller/Disturbance Estimator/getx ==
  q : Inport
  qdot : Inport  Port=2
  H : Inport  Port=3
  Demux : Demux  Outputs=2
  Demux1 : Demux  Outputs=2
  Discrete Derivative : simulink/Discrete/Discrete Derivative  gainval=1.0  ICPrevScaledInput=0.0  InputProcessing=Inherited  OutMin=[]  OutMax=[]  OutDataType=fixdt(1, 16)  OutScaling=2^-10  RndMeth=Round  DoSatur=off
  Mux : Mux
  Product6 : Product  Multiplication=Matrix(*)  RndMeth=Zero
  Reshape : Reshape  OutputDimensionality=Column vector (2-D)
  x : Outport
  xdot : Outport  Port=2
  wires:
  Discrete Derivative/1 -> xdot/1  "xdot"
  q/1 -> [q]
  qdot/1 -> [qdot]
  H/1 -> [H]
  [H] -> Product6/1
  [qdot] -> Product6/2
  [q] -> Demux/1
  Product6/1 -> Demux1/1
  Demux/1 -> Mux/1
  Demux/2 -> Mux/2
  Demux1/1 -> Mux/3
  Demux1/2 -> Mux/4
  Mux/1 -> Reshape/1
  Reshape/1 -> x/1, Discrete Derivative/1

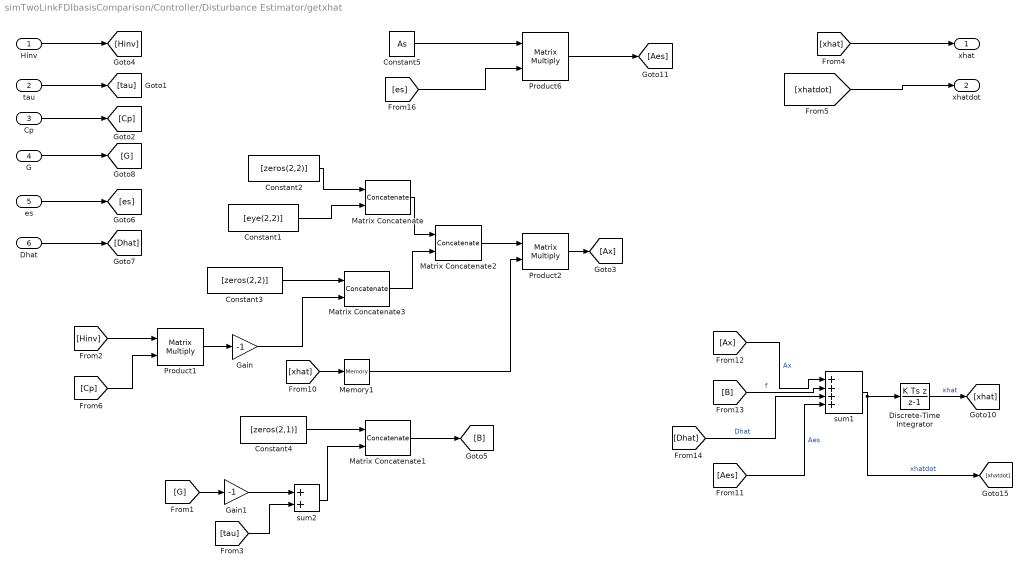
== system simTwoLinkFDIbasisComparison/Controller/Disturbance Estimator/getxhat ==
  Hinv : Inport
  tau : Inport  Port=2
  Cp : Inport  Port=3
  G : Inport  Port=4
  es : Inport  Port=5
  Dhat : Inport  Port=6
  Constant1 : Constant  Value=[eye(2,2)]  VectorParams1D=off
  Constant2 : Constant  Value=[zeros(2,2)]  VectorParams1D=off
  Constant3 : Constant  Value=[zeros(2,2)]
  Constant4 : Constant  Value=[zeros(2,1)]  VectorParams1D=off
  Constant5 : Constant  Value=As
  Discrete-Time Integrator : DiscreteIntegrator  IntegratorMethod=Integration: Backward Euler  InitialCondition=xhat0  InitialConditionSetting=State (most efficient)  SampleTime=-1  UpperSaturationLimit=Intmax  LowerSaturationLimit=Intmin
  Gain : Gain  Gain=-1
  Gain1 : Gain  Gain=-1
  Matrix Concatenate : Concatenate  Mode=Multidimensional array  ConcatenateDimension=2
  Matrix Concatenate1 : Concatenate  Mode=Multidimensional array
  Matrix Concatenate2 : Concatenate  Mode=Multidimensional array
  Matrix Concatenate3 : Concatenate  Mode=Multidimensional array  ConcatenateDimension=2
  Memory1 : Memory  X0=xhat0  InheritSampleTime=on  LinearizeMemory=on  LinearizeAsDelay=on
  Product1 : Product  Multiplication=Matrix(*)  RndMeth=Zero
  Product2 : Product  Multiplication=Matrix(*)  RndMeth=Zero
  Product6 : Product  Multiplication=Matrix(*)  RndMeth=Zero
  sum1 : Sum  Inputs=++++
  sum2 : Sum
  xhat : Outport
  xhatdot : Outport  Port=2
  wires:
  [Dhat] -> sum1/3  "Dhat"
  [B] -> sum1/2  "f"
  [Ax] -> sum1/1  "Ax"
  [Aes] -> sum1/4  "Aes"
  sum1/1 -> [xhatdot], Discrete-Time Integrator/1  "xhatdot"
  Discrete-Time Integrator/1 -> [xhat]  "xhat"
  Memory1/1 -> Product2/2
  Product2/1 -> [Ax]
  [xhat] -> Memory1/1
  Matrix Concatenate/1 -> Matrix Concatenate2/1
  Constant2/1 -> Matrix Concatenate/1
  Hinv/1 -> [Hinv]
  Matrix Concatenate2/1 -> Product2/1
  tau/1 -> [tau]
  Cp/1 -> [Cp]
  [G] -> Gain1/1
  [tau] -> sum2/2
  Constant4/1 -> Matrix Concatenate1/1
  sum2/1 -> Matrix Concatenate1/2
  Matrix Concatenate1/1 -> [B]
  Product6/1 -> [Aes]
  Constant5/1 -> Product6/1
  [es] -> Product6/2
  es/1 -> [es]
  Dhat/1 -> [Dhat]
  G/1 -> [G]
  Constant1/1 -> Matrix Concatenate/2
  Constant3/1 -> Matrix Concatenate3/1
  Matrix Concatenate3/1 -> Matrix Concatenate2/2
  [Hinv] -> Product1/1
  [Cp] -> Product1/2
  Product1/1 -> Gain/1
  Gain/1 -> Matrix Concatenate3/2
  Gain1/1 -> sum2/1
  [xhat] -> xhat/1
  [xhatdot] -> xhatdot/1

== system simTwoLinkFDIbasisComparison/Controller/Get System Parameters/Energy Calculation ==
  q : Inport
  qdot : Inport  Port=2
  H : Inport  Port=3
  Constant : Constant  Value=l1  VectorParams1D=off
  Constant1 : Constant  Value=l2  VectorParams1D=off
  Demux : Demux  Outputs=2
  Gain : Gain  Gain=1/2
  Gain1 : Gain  Gain=0.5
  Gain5 : Gain  Gain=0.5*m1*g
  Gain6 : Gain  Gain=m2*g
  Math Function : Math  Operator=transpose  SaturateOnIntegerOverflow=on
  Product1 : Product  RndMeth=Zero
  Product3 : Product  RndMeth=Zero
  Product5 : Product  Inputs=3  Multiplication=Matrix(*)  RndMeth=Zero
  Sum of Elements : Sum  Inputs=+
  Sum1 : Sum
  Sum2 : Sum
  Sum3 : Sum
  Terminator4 : Terminator
  Trigonometric Function : Trigonometry
  Trigonometric Function2 : Trigonometry
  U : Outport
  T : Outport  Port=2
  E : Outport  Port=3
  wires:
  [q] -> Trigonometric Function/1, Sum of Elements/1
  Trigonometric Function/1 -> Demux/1
  Demux/1 -> [s1]
  Demux/2 -> Terminator4/1
  Sum of Elements/1 -> Trigonometric Function2/1
  Trigonometric Function2/1 -> [s12]
  [qdot] -> Math Function/1
  Math Function/1 -> Product5/1
  [H] -> Product5/2
  [qdot] -> Product5/3
  Product5/1 -> Gain/1
  [l1sintht1] -> Gain5/1
  Gain/1 -> [T]
  [l1sintht1] -> Sum1/1
  [l2sintht12] -> Gain1/1
  Gain5/1 -> Sum3/1
  Gain6/1 -> Sum3/2
  [T] -> Sum2/1
  [U] -> Sum2/2
  q/1 -> [q]
  qdot/1 -> [qdot]
  Sum2/1 -> E/1  "E"
  [U] -> U/1  "U"
  [T] -> T/1  "T"
  Constant/1 -> Product1/1
  [s1] -> Product1/2
  Product1/1 -> [l1sintht1]
  Constant1/1 -> Product3/1
  [s12] -> Product3/2
  Product3/1 -> [l2sintht12]
  Gain1/1 -> Sum1/2
  Sum1/1 -> Gain6/1
  Sum3/1 -> [U]
  H/1 -> [H]

== system simTwoLinkFDIbasisComparison/Controller/Get System Parameters/get Plant Parameters ==
  H : Inport
  C : Inport  Port=2
  G : Inport  Port=3
  qdot : Inport  Port=4
  Cprime : Inport  Port=5
  {1,5,7,11} (4 alike) : Selector  NumberOfDimensions=2  InputPortWidth=3  IndexOptions=Index vector (dialog),Index vector (dialog)  Indices=1,1  OutputSizes=1,1
  12 : Selector  NumberOfDimensions=2  InputPortWidth=3  IndexOptions=Index vector (dialog),Index vector (dialog)  Indices=1,2  OutputSizes=1,1
  2 : Selector  NumberOfDimensions=2  InputPortWidth=3  IndexOptions=Index vector (dialog),Index vector (dialog)  Indices=1,2  OutputSizes=1,1
  {3,6,8,21} (4 alike) : Selector  NumberOfDimensions=2  InputPortWidth=3  IndexOptions=Index vector (dialog),Index vector (dialog)  Indices=2,1  OutputSizes=1,1
  22 : Selector  NumberOfDimensions=2  InputPortWidth=3  IndexOptions=Index vector (dialog),Index vector (dialog)  Indices=2,2  OutputSizes=1,1
  4 : Selector  NumberOfDimensions=2  InputPortWidth=3  IndexOptions=Index vector (dialog),Index vector (dialog)  Indices=2,2  OutputSizes=1,1
  Bus Creator : BusCreator  Inputs=16
  Product5 : Product  Multiplication=Matrix(*)  RndMeth=Zero
  Sum of Elements1 : Sum
  busData : Outport
  wires:
  [H] -> 11/1, 12/1, 21/1, 22/1
  [C] -> 1/1, 2/1, 4/1, 3/1
  [G] -> 6/1, 5/1
  [C] -> Product5/1
  [qdot] -> Product5/2
  Product5/1 -> Sum of Elements1/1
  [G] -> Sum of Elements1/2
  Sum of Elements1/1 -> 7/1, 8/1
  Bus Creator/1 -> busData/1
  H/1 -> [H]  "H"
  C/1 -> [C]  "C"
  G/1 -> [G]  "G"
  qdot/1 -> [qdot]
  [G] -> Bus Creator/4
  [Cprime] -> Bus Creator/3
  [C] -> Bus Creator/2
  [H] -> Bus Creator/1
  22/1 -> Bus Creator/8  "H22"
  21/1 -> Bus Creator/7  "H21"
  1/1 -> Bus Creator/9  "C11"
  12/1 -> Bus Creator/6  "H12"
  2/1 -> Bus Creator/10  "C12"
  11/1 -> Bus Creator/5  "H11"
  3/1 -> Bus Creator/11  "C21"
  4/1 -> Bus Creator/12  "C22"
  5/1 -> Bus Creator/13  "G_1"
  6/1 -> Bus Creator/14  "G_2"
  7/1 -> Bus Creator/15  "phi1"
  8/1 -> Bus Creator/16  "phi2"
  Cprime/1 -> [Cprime]  "Cprime"

== system simTwoLinkFDIbasisComparison/Controller/Get System Parameters/getC ==
  s2 : Inport
  q1dot : Inport  Port=2
  q2dot : Inport  Port=3
  m2 : Inport  Port=4
  Constant2 : Constant  Value=0  VectorParams1D=off
  Gain4 : Gain  Gain=l1*lc2
  Gain6 : Gain  Gain=-1
  Gain7 : Gain  Gain=-1
  Matrix Concatenate : Concatenate  Mode=Multidimensional array  ConcatenateDimension=2
  Matrix Concatenate1 : Concatenate  Mode=Multidimensional array  ConcatenateDimension=2
  Matrix Concatenate2 : Concatenate  Mode=Multidimensional array
  Product{,8..10} (4 alike) : Product  RndMeth=Zero
  Sum4 : Sum
  C : Outport
  wires:
  s2/1 -> [s2]
  q1dot/1 -> [q1dot]
  q2dot/1 -> [q2dot]
  [C] -> C/1
  [m2] -> Gain4/1
  Gain4/1 -> Product/1
  [s2] -> Product/2
  Product/1 -> [h]
  [h] -> Gain6/1
  [h] -> Gain7/1
  Sum4/1 -> Product10/1
  Gain7/1 -> Product10/2
  Product10/1 -> [C12]
  [q2dot] -> Sum4/2
  Constant2/1 -> [C22]
  [h] -> Product8/2
  [q1dot] -> Product8/1
  Product8/1 -> [C21]
  Gain6/1 -> Product9/2
  Product9/1 -> [C11]
  [q2dot] -> Product9/1
  [q1dot] -> Sum4/1
  Matrix Concatenate2/1 -> [C]
  [C22] -> Matrix Concatenate1/2
  [C21] -> Matrix Concatenate1/1
  Matrix Concatenate1/1 -> Matrix Concatenate2/2
  Matrix Concatenate/1 -> Matrix Concatenate2/1
  [C12] -> Matrix Concatenate/2
  [C11] -> Matrix Concatenate/1
  m2/1 -> [m2]

== system simTwoLinkFDIbasisComparison/Controller/Get System Parameters/getCprime ==
  s2 : Inport
  q1dot : Inport  Port=2
  q2dot : Inport  Port=3
  Constant1 : Constant  Value=0  VectorParams1D=off
  Constant2 : Constant  Value=m2
  Gain1 : Gain  Gain=2
  Gain2 : Gain  Gain=l1*lc2
  Gain4 : Gain  Gain=-1
  Gain6 : Gain  Gain=-3
  Gain7 : Gain  Gain=-1
  Matrix Concatenate : Concatenate  Mode=Multidimensional array  ConcatenateDimension=2
  Matrix Concatenate1 : Concatenate  Mode=Multidimensional array  ConcatenateDimension=2
  Matrix Concatenate2 : Concatenate  Mode=Multidimensional array
  Product{,1,9..10} (4 alike) : Product  RndMeth=Zero
  Sum1 : Sum  Inputs=-+
  Sum4 : Sum
  Cprime : Outport
  wires:
  s2/1 -> [s2]
  q1dot/1 -> [q1dot]
  q2dot/1 -> [q2dot]
  [h] -> Gain6/1
  [h] -> Gain7/1
  Sum4/1 -> Product10/1
  Gain7/1 -> Product10/2
  Product10/1 -> [C12]
  [q2dot] -> Gain1/1
  Constant1/1 -> [C22]
  Gain6/1 -> Product9/2
  Product9/1 -> [C11]
  [q2dot] -> Product9/1
  [q1dot] -> Sum4/1
  Matrix Concatenate2/1 -> Cprime/1
  [C22] -> Matrix Concatenate1/2
  [C21] -> Matrix Concatenate1/1
  Matrix Concatenate1/1 -> Matrix Concatenate2/2
  Matrix Concatenate/1 -> Matrix Concatenate2/1
  [C12] -> Matrix Concatenate/2
  [C11] -> Matrix Concatenate/1
  Gain1/1 -> Sum4/2
  [h] -> Gain4/1
  Sum1/1 -> Product1/1
  Gain4/1 -> Product1/2
  Product1/1 -> [C21]
  [q2dot] -> Sum1/2
  [q1dot] -> Sum1/1
  [m2] -> Gain2/1
  Gain2/1 -> Product/1
  [s2] -> Product/2
  Product/1 -> [h]
  Constant2/1 -> [m2]

== system simTwoLinkFDIbasisComparison/Controller/Get System Parameters/getG ==
  c1 : Inport
  c12 : Inport  Port=2
  m1 : Inport  Port=3
  m2 : Inport  Port=4
  Add1 : Sum
  Add2 : Sum
  Gain10 : Gain  Gain=lc2
  Gain11 : Gain  Gain=g
  Gain2 : Gain
  Gain5 : Gain  Gain=lc1
  Gain6 : Gain  Gain=l1
  Gain7 : Gain  Gain=g
  Gain8 : Gain  Gain=lc2
  Gain9 : Gain  Gain=g
  Matrix Concatenate2 : Concatenate  Mode=Multidimensional array
  Product1 : Product  RndMeth=Zero
  Product2 : Product  RndMeth=Zero
  Product3 : Product  RndMeth=Zero
  G : Outport
  wires:
  c12/1 -> [c12]
  c1/1 -> [c1]
  Matrix Concatenate2/1 -> Gain2/1
  [G11] -> Matrix Concatenate2/1
  [G21] -> Matrix Concatenate2/2
  Gain2/1 -> G/1
  [m1] -> Gain5/1
  Gain5/1 -> Add1/1
  [m2] -> Gain6/1
  Gain6/1 -> Add1/2
  Add1/1 -> Gain7/1
  Gain7/1 -> Product1/1
  [c1] -> Product1/2
  [m2] -> Gain8/1
  Gain8/1 -> Gain9/1
  Gain9/1 -> Product2/1
  [c12] -> Product2/2
  Product1/1 -> Add2/1
  Product2/1 -> Add2/2
  Add2/1 -> [G11]
  [m2] -> Gain10/1
  Gain10/1 -> Gain11/1
  Gain11/1 -> Product3/1
  [c12] -> Product3/2
  Product3/1 -> [G21]
  m1/1 -> [m1]
  m2/1 -> [m2]

== system simTwoLinkFDIbasisComparison/Controller/Get System Parameters/getH ==
  c2 : Inport
  m1 : Inport  Port=2
  m2 : Inport  Port=3
  Constant2 : Constant  Value=I2
  Constant4 : Constant  Value=I1
  Gain : Gain  Gain=2
  Gain1 : Gain  Gain=lc2^2
  Gain4 : Gain  Gain=l1*lc2
  Gain5 : Gain  Gain=lc1^2
  Gain6 : Gain  Gain=l1^2+lc2^2
  Gain7 : Gain  Gain=lc2^2
  Matrix Concatenate : Concatenate  Mode=Multidimensional array  ConcatenateDimension=2
  Matrix Concatenate1 : Concatenate  Mode=Multidimensional array  ConcatenateDimension=2
  Matrix Concatenate2 : Concatenate  Mode=Multidimensional array
  Product : Product  RndMeth=Zero
  Sum : Sum  Inputs=+++++
  Sum1 : Sum  Inputs=+++
  Sum2 : Sum
  H : Outport
  wires:
  [H11] -> Matrix Concatenate/1
  [H12] -> Matrix Concatenate/2
  Matrix Concatenate/1 -> Matrix Concatenate2/1
  Matrix Concatenate1/1 -> Matrix Concatenate2/2
  [H21] -> Matrix Concatenate1/1
  [H22] -> Matrix Concatenate1/2
  Matrix Concatenate2/1 -> H/1
  c2/1 -> [c2]
  Sum/1 -> [H11]
  Sum1/1 -> [H12], [H21]
  [m2] -> Gain4/1
  Gain4/1 -> Product/1
  [c2] -> Product/2
  Product/1 -> [a]
  [m1] -> Gain5/1
  [m2] -> Gain6/1
  [I1] -> Sum/1
  [I2] -> Sum/2
  Gain5/1 -> Sum/3
  [a] -> Gain/1
  Gain6/1 -> Sum/4
  Gain/1 -> Sum/5
  [m2] -> Gain7/1
  [I2] -> Sum1/1
  Gain7/1 -> Sum1/2
  [a] -> Sum1/3
  [m2] -> Gain1/1
  [I2] -> Sum2/1
  Gain1/1 -> Sum2/2
  Sum2/1 -> [H22]
  Constant4/1 -> [I1]
  Constant2/1 -> [I2]
  m1/1 -> [m1]
  m2/1 -> [m2]

== system simTwoLinkFDIbasisComparison/Controller/Nominal Controller/FBL Controller ==
  r : Inport
  q : Inport  Port=2
  qdot : Inport  Port=3
  H : Inport  Port=4
  Phi : Inport  Port=5
  Add : Sum  Inputs=-+
  Add1 : Sum  Inputs=-+
  Add2 : Sum
  Add3 : Sum
  Add4 : Sum
  Constant2 : Constant  Value=[0 0]'
  Discrete Derivative : simulink/Discrete/Discrete Derivative  gainval=1.0  ICPrevScaledInput=0.0  InputProcessing=Inherited  OutMin=[]  OutMax=[]  OutDataType=fixdt(1, 16)  OutScaling=2^-10  DoSatur=off
  Gain : Gain  Gain=-Kv
  Gain1 : Gain  Gain=-Kp
  Product2 : Product  Multiplication=Matrix(*)  RndMeth=Zero
  Saturation : Saturate  UpperLimit=10  LowerLimit=-10
  tau : Outport
  wires:
  [v] -> Product2/2
  Product2/1 -> Add4/1
  [Phi] -> Add4/2
  [H] -> Product2/1
  [r] -> Add/1
  Add/1 -> [e]  "e"
  Discrete Derivative/1 -> Saturation/1
  [qdot] -> Add1/2
  Add1/1 -> [edot]  "edot"
  [edot] -> Gain/1
  Constant2/1 -> Add2/1
  Gain/1 -> Add2/2
  [e] -> Gain1/1
  Add2/1 -> Add3/1
  Gain1/1 -> Add3/2
  Add3/1 -> [v]  "v"
  [q] -> Add/2
  [r] -> Discrete Derivative/1
  Saturation/1 -> Add1/1
  r/1 -> [r]  "r"
  Phi/1 -> [Phi]
  H/1 -> [H]
  Add4/1 -> tau/1  "tau"
  q/1 -> [q]
  qdot/1 -> [qdot]

== system simTwoLinkFDIbasisComparison/System/System Parameters/Energy Calculation ==
  q : Inport
  qdot : Inport  Port=2
  H : Inport  Port=3
  Constant : Constant  Value=l1  VectorParams1D=off
  Constant1 : Constant  Value=l2  VectorParams1D=off
  Demux : Demux  Outputs=2
  Gain : Gain  Gain=1/2
  Gain1 : Gain  Gain=0.5
  Gain5 : Gain  Gain=0.5*m1*g
  Gain6 : Gain  Gain=m2*g
  Math Function : Math  Operator=transpose  SaturateOnIntegerOverflow=on
  Product1 : Product  RndMeth=Zero
  Product3 : Product  RndMeth=Zero
  Product5 : Product  Inputs=3  Multiplication=Matrix(*)  RndMeth=Zero
  Sum of Elements : Sum  Inputs=+
  Sum1 : Sum
  Sum2 : Sum
  Sum3 : Sum
  Terminator4 : Terminator
  Trigonometric Function : Trigonometry
  Trigonometric Function2 : Trigonometry
  U : Outport
  T : Outport  Port=2
  E : Outport  Port=3
  wires:
  [q] -> Trigonometric Function/1, Sum of Elements/1
  Trigonometric Function/1 -> Demux/1
  Demux/1 -> [s1]
  Demux/2 -> Terminator4/1
  Sum of Elements/1 -> Trigonometric Function2/1
  Trigonometric Function2/1 -> [s12]
  [qdot] -> Math Function/1
  Math Function/1 -> Product5/1
  [H] -> Product5/2
  [qdot] -> Product5/3
  Product5/1 -> Gain/1
  [l1sintht1] -> Gain5/1
  Gain/1 -> [T]
  [l1sintht1] -> Sum1/1
  [l2sintht12] -> Gain1/1
  Gain5/1 -> Sum3/1
  Gain6/1 -> Sum3/2
  [T] -> Sum2/1
  [U] -> Sum2/2
  q/1 -> [q]
  qdot/1 -> [qdot]
  Sum2/1 -> E/1  "E"
  [U] -> U/1  "U"
  [T] -> T/1  "T"
  Constant/1 -> Product1/1
  [s1] -> Product1/2
  Product1/1 -> [l1sintht1]
  Constant1/1 -> Product3/1
  [s12] -> Product3/2
  Product3/1 -> [l2sintht12]
  Gain1/1 -> Sum1/2
  Sum1/1 -> Gain6/1
  Sum3/1 -> [U]
  H/1 -> [H]

== system simTwoLinkFDIbasisComparison/System/System Parameters/get Plant Parameters ==
  H : Inport
  C : Inport  Port=2
  G : Inport  Port=3
  qdot : Inport  Port=4
  {1,5,7,11} (4 alike) : Selector  NumberOfDimensions=2  InputPortWidth=3  IndexOptions=Index vector (dialog),Index vector (dialog)  Indices=1,1  OutputSizes=1,1
  12 : Selector  NumberOfDimensions=2  InputPortWidth=3  IndexOptions=Index vector (dialog),Index vector (dialog)  Indices=1,2  OutputSizes=1,1
  2 : Selector  NumberOfDimensions=2  InputPortWidth=3  IndexOptions=Index vector (dialog),Index vector (dialog)  Indices=1,2  OutputSizes=1,1
  {3,6,8,21} (4 alike) : Selector  NumberOfDimensions=2  InputPortWidth=3  IndexOptions=Index vector (dialog),Index vector (dialog)  Indices=2,1  OutputSizes=1,1
  22 : Selector  NumberOfDimensions=2  InputPortWidth=3  IndexOptions=Index vector (dialog),Index vector (dialog)  Indices=2,2  OutputSizes=1,1
  4 : Selector  NumberOfDimensions=2  InputPortWidth=3  IndexOptions=Index vector (dialog),Index vector (dialog)  Indices=2,2  OutputSizes=1,1
  Bus Creator : BusCreator  Inputs=15
  Product5 : Product  Multiplication=Matrix(*)  RndMeth=Zero
  Sum of Elements1 : Sum
  busData : Outport
  wires:
  2/1 -> Bus Creator/9  "C12"
  21/1 -> Bus Creator/6  "H21"
  22/1 -> Bus Creator/7  "H22"
  4/1 -> Bus Creator/11  "C22"
  6/1 -> Bus Creator/13  "G_2"
  1/1 -> Bus Creator/8  "C11"
  5/1 -> Bus Creator/12  "G_1"
  12/1 -> Bus Creator/5  "H12"
  3/1 -> Bus Creator/10  "C21"
  11/1 -> Bus Creator/4  "H11"
  [H] -> 11/1, 12/1, 21/1, 22/1
  [C] -> 1/1, 2/1, 4/1, 3/1
  [G] -> 6/1, 5/1
  [C] -> Product5/1
  [qdot] -> Product5/2
  Product5/1 -> Sum of Elements1/1
  [G] -> Sum of Elements1/2
  Sum of Elements1/1 -> 7/1, 8/1
  7/1 -> Bus Creator/14  "phi1"
  8/1 -> Bus Creator/15  "phi2"
  [G] -> Bus Creator/3
  Bus Creator/1 -> busData/1
  [C] -> Bus Creator/2
  [H] -> Bus Creator/1
  H/1 -> [H]  "H"
  C/1 -> [C]  "C"
  G/1 -> [G]  "G"
  qdot/1 -> [qdot]

== system simTwoLinkFDIbasisComparison/System/System Parameters/getC ==
  s2 : Inport
  q1dot : Inport  Port=2
  q2dot : Inport  Port=3
  m2 : Inport  Port=4
  Add : Sum
  Constant2 : Constant  Value=c2  VectorParams1D=off
  Constant3 : Constant  Value=c1  VectorParams1D=off
  Gain4 : Gain  Gain=l1*lc2
  Gain6 : Gain  Gain=-1
  Gain7 : Gain  Gain=-1
  Matrix Concatenate : Concatenate  Mode=Multidimensional array  ConcatenateDimension=2
  Matrix Concatenate1 : Concatenate  Mode=Multidimensional array  ConcatenateDimension=2
  Matrix Concatenate2 : Concatenate  Mode=Multidimensional array
  Product{,8..10} (4 alike) : Product  RndMeth=Zero
  Sum4 : Sum
  C : Outport
  wires:
  s2/1 -> [s2]
  q1dot/1 -> [q1dot]
  q2dot/1 -> [q2dot]
  [C] -> C/1
  [m2] -> Gain4/1
  Gain4/1 -> Product/1
  [s2] -> Product/2
  Product/1 -> [h]
  [h] -> Gain6/1
  [h] -> Gain7/1
  Sum4/1 -> Product10/1
  Gain7/1 -> Product10/2
  Product10/1 -> [C12]
  [q2dot] -> Sum4/2
  Constant2/1 -> [C22]
  [h] -> Product8/2
  [q1dot] -> Product8/1
  Product8/1 -> [C21]
  Gain6/1 -> Product9/2
  [q2dot] -> Product9/1
  [q1dot] -> Sum4/1
  Matrix Concatenate2/1 -> [C]
  [C22] -> Matrix Concatenate1/2
  [C21] -> Matrix Concatenate1/1
  Matrix Concatenate1/1 -> Matrix Concatenate2/2
  Matrix Concatenate/1 -> Matrix Concatenate2/1
  [C12] -> Matrix Concatenate/2
  [C11] -> Matrix Concatenate/1
  Product9/1 -> Add/1
  Constant3/1 -> Add/2
  Add/1 -> [C11]
  m2/1 -> [m2]

== system simTwoLinkFDIbasisComparison/System/System Parameters/getG ==
  c1 : Inport
  c12 : Inport  Port=2
  m1 : Inport  Port=3
  m2 : Inport  Port=4
  Add1 : Sum
  Add2 : Sum
  Gain10 : Gain  Gain=lc2
  Gain11 : Gain  Gain=g
  Gain5 : Gain  Gain=lc1
  Gain6 : Gain  Gain=l1
  Gain7 : Gain  Gain=g
  Gain8 : Gain  Gain=lc2
  Gain9 : Gain  Gain=g
  Matrix Concatenate2 : Concatenate  Mode=Multidimensional array
  Product1 : Product  RndMeth=Zero
  Product2 : Product  RndMeth=Zero
  Product3 : Product  RndMeth=Zero
  G : Outport
  wires:
  c12/1 -> [c12]
  c1/1 -> [c1]
  Matrix Concatenate2/1 -> G/1
  [G11] -> Matrix Concatenate2/1
  [G21] -> Matrix Concatenate2/2
  [m1] -> Gain5/1
  Gain5/1 -> Add1/1
  [m2] -> Gain6/1
  Gain6/1 -> Add1/2
  Add1/1 -> Gain7/1
  Gain7/1 -> Product1/1
  [c1] -> Product1/2
  [m2] -> Gain8/1
  Gain8/1 -> Gain9/1
  Gain9/1 -> Product2/1
  [c12] -> Product2/2
  Product1/1 -> Add2/1
  Product2/1 -> Add2/2
  Add2/1 -> [G11]
  [m2] -> Gain10/1
  Gain10/1 -> Gain11/1
  Gain11/1 -> Product3/1
  [c12] -> Product3/2
  Product3/1 -> [G21]
  m1/1 -> [m1]
  m2/1 -> [m2]
